simulink model "bangbangthermostat"  (R2020a)
settings: Solver=VariableStepAuto  StartTime=0.0  StopTime=10.0  RelTol=1e-3
PreLoadFcn:
  | k=0.5
InitFcn:
  | k=0.5
settings Model: Creator=jyotirmoy  LastModifiedBy=jyotirmoy

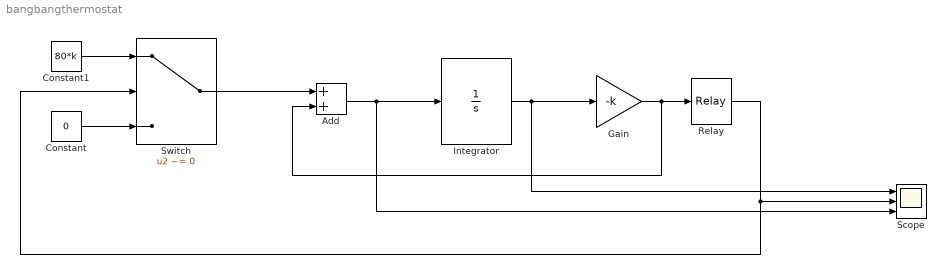
== system bangbangthermostat ==
  Add : Sum
  Constant : Constant  Value=0
  Constant1 : Constant  Value=80*k
  Gain : Gain  Gain=-k
  Integrator : Integrator  InitialCondition=72
  Relay : Relay  OnSwitchValue=-70*k  OffSwitchValue=-75*k
  Scope : Scope  NumInputPorts=3
  Switch : Switch  Criteria=u2 ~= 0
  wires:
  Integrator/1 -> Gain/1, Scope/1
  Switch/1 -> Add/1
  Constant1/1 -> Switch/1
  Constant/1 -> Switch/3
  Add/1 -> Scope/3, Integrator/1
  Relay/1 -> Switch/2, Scope/2
  Gain/1 -> Add/2, Relay/1
